simulink model "UAM_controller"  (R2024b)
settings: Solver=FixedStepAuto  StartTime=0.0  StopTime=10.0  RelTol=1e-3
undefined symbols (not defined in the file): control, controlParams, ControlSampleTime, Cruise_a, DiscIntNeverNeededParam, flightState, FWControlParams, FWTrimSpeed, uavParam, w_trim
libraries: slpidlib x41, simulink x7
(part 1 of 6)
settings Model: DataDictionary=UAM_data.sldd  Creator=admin  LastModifiedBy=admin
settings OptimizationCC: DefaultParameterBehavior=Inlined  EnhancedBackFolding=on  PassReuseOutputArgsAs=Individual arguments  ZeroExternalMemoryAtStartup=off  ZeroInternalMemoryAtStartup=off  OptimizeBlockOrder=speed  DifferentSizesBufferReuse=on  OptimizationCustomize=off  EfficientTunableParamExpr=on
settings DebuggingCC: ParameterTunabilityLossMsg=error
settings HardwareCC: ProdBitPerLong=64  ProdLargestAtomicInteger=LongLong  ProdLargestAtomicFloat=Double  ProdLongLongMode=on  ProdHWDeviceType=ARM Compatible->ARM Cortex-A (64-bit)
settings SFSimCC: MATLABDynamicMemAlloc=off
settings RTWCC: Description=Embedded Coder  SystemTargetFile=ert.tlc  TemplateMakefile=ert_default_tmf  Toolchain=Linaro AArch64 Linux v6.3.1
settings CodeAppCC: ForceParamTrailComments=on  IgnoreCustomStorageClasses=off  OperatorAnnotations=on  SimulinkDataObjDesc=on  SFDataObjDesc=on  CustomSymbolStrGlobalVar=CTRL_$N$M  CustomSymbolStrType=CTRL_$N$M_T  CustomSymbolStrField=CTRL_$N$M  CustomSymbolStrFcn=CTRL_$N$M$F  CustomSymbolStrBlkIO=CTRL_rtb_$N$M  CustomSymbolStrTmpVar=CTRL_tmp_$N$M  CustomSymbolStrMacro=CTRL_$N$M_MACRO  InsertBlockDesc=on
settings ERTTargetCC: TargetLangStandard=C99 (ISO)  GenerateSampleERTMain=on  ERTCustomFileTemplate=example_file_process.tlc

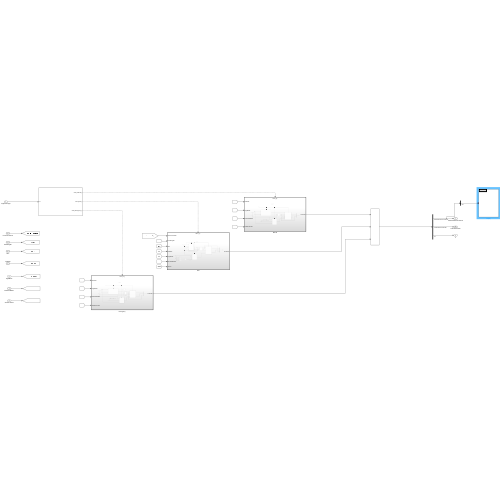
[thumbnail: Simulink's stored preview of the top-level diagram]
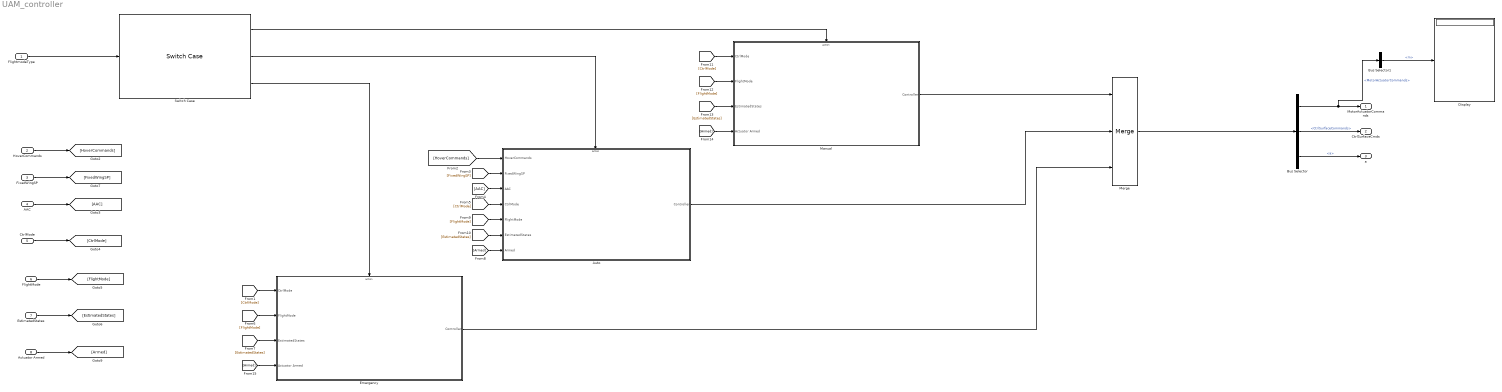
== system UAM_controller ==
  FlightmodeType : Inport  OutDataTypeStr=Enum: FlightModeType
  HoverCommands : Inport  Port=2  OutDataTypeStr=Bus: HoverSPBus
  FixedWingSP : Inport  Port=3  OutDataTypeStr=Bus: FixedWingCommandBus
  AAC : Inport  Port=4  OutDataTypeStr=Bus: AAC
  CtrlMode : Inport  Port=5  OutDataTypeStr=Bus: controlMode
  FlightMode : Inport  Port=6
  EstimatedStates : Inport  Port=7  OutDataTypeStr=Bus: StateBus
  Actuator Armed : Inport  Port=8
  Auto : Subsystem  TreatAsAtomicUnit=on
  Bus Selector : BusSelector  OutputSignals=MotorActuatorCommands,CtrlSurfaceCommands,a
  Bus Selector1 : BusSelector  OutputSignals=m
  Display : Display
  Emergency : Subsystem  TreatAsAtomicUnit=on
  Manual : Subsystem  TreatAsAtomicUnit=on
  Merge : Merge  Inputs=3
  Switch Case : SwitchCase  CaseConditions={FlightModeType.Manual, FlightModeType.Auto, FlightModeType.Emergecny}  ShowDefaultCase=off
  MotorActuatorCommands : Outport  OutDataTypeStr=Bus: FCCData
  CtrlSurfaceCmds : Outport  Port=2  OutDataTypeStr=Bus: FixedWingCtrlBus
  a : Outport  Port=3
  wires:
  FlightmodeType/1 -> Switch Case/1
  CtrlMode/1 -> [CtrlMode]
  HoverCommands/1 -> [HoverCommands]
  EstimatedStates/1 -> [EstimatedStates]
  FlightMode/1 -> [FlightMode]
  AAC/1 -> [AAC]
  FixedWingSP/1 -> [FixedWingSP]
  Actuator Armed/1 -> [Armed]
  [FlightMode] -> Auto/5(FlightMode)
  [Armed] -> Auto/7(" Armed")
  [EstimatedStates] -> Auto/6(EstimatedStates)
  [CtrlMode] -> Auto/4(CtrlMode)
  [AAC] -> Auto/3(AAC)
  [FixedWingSP] -> Auto/2(FixedWingSP)
  [HoverCommands] -> Auto/1(HoverCommands)
  Switch Case/2 -> Auto/Action
  Switch Case/1 -> Manual/Action
  [CtrlMode] -> Manual/1(CtrlMode)
  [FlightMode] -> Manual/2(FlightMode)
  [EstimatedStates] -> Manual/3(EstimatedStates)
  [Armed] -> Manual/4(Actuator Armed)
  [Armed] -> Emergency/4(Actuator Armed)
  [FlightMode] -> Emergency/2(FlightMode)
  [EstimatedStates] -> Emergency/3(EstimatedStates)
  [CtrlMode] -> Emergency/1(CtrlMode)
  Switch Case/3 -> Emergency/Action
  Manual/1(Controller) -> Merge/1
  Merge/1 -> Bus Selector/1
  Bus Selector/1 -> Bus Selector1/1, MotorActuatorCommands/1  "<MotorActuatorCommands>"
  Bus Selector/2 -> CtrlSurfaceCmds/1  "<CtrlSurfaceCommands>"
  Bus Selector/3 -> a/1  "<a>"
  Auto/1(Controller) -> Merge/2
  Emergency/1(Controller) -> Merge/3
  Bus Selector1/1 -> Display/1  "<m>"

== system UAM_controller/Auto ==
  HoverCommands : Inport  OutDataTypeStr=Bus: HoverSPBus
  FixedWingSP : Inport  Port=2
  AAC : Inport  Port=3
  CtrlMode : Inport  Port=4
  FlightMode : Inport  Port=5
  EstimatedStates : Inport  Port=6
  " Armed" : Inport  Port=7
  Action Port : ActionPort  ActionPortLabel=case [ 1 ]:
  Blend Scheduler : Subsystem
  Bus Creator : BusCreator  Inputs=3  OutDataTypeStr=Bus: controller
  Bus Selector2 : BusSelector  OutputSignals=inTransition,TransitionCondition,BackTransitionCondition,TransitionStep
  Fixed Wing Controller : Subsystem  TreatAsAtomicUnit=on  VariantControl=Fixed Wing Controller
  Manual Control : Subsystem
  Multicopter Controller : Subsystem  TreatAsAtomicUnit=on
  Scheduler : Subsystem  SystemSampleTime=0.005
  Controller : Outport
  wires:
  Scheduler/1(MotorActuatorCommands) -> Bus Creator/1  "MotorActuatorCommands"
  Manual Control/1(AERT) -> Fixed Wing Controller/5(AERT)
  Scheduler/2(CtrlSurfaceCommands) -> Bus Creator/2  "CtrlSurfaceCommands"
  Fixed Wing Controller/1(Actuator) -> Scheduler/3(FixedWingActuators)
  Blend Scheduler/2(alpha) -> Bus Creator/3  "a"
  Multicopter Controller/1(MixerCommands) -> Blend Scheduler/3(MixerCommands)
  AAC/1 -> Fixed Wing Controller/3(AAC SP)
  FixedWingSP/1 -> Fixed Wing Controller/4(FixedWingSP)
  [InTransition] -> Multicopter Controller/3(InTransition)
  " Armed"/1 -> Fixed Wing Controller/Enable, Scheduler/Enable, Multicopter Controller/Enable
  HoverCommands/1 -> Multicopter Controller/1(Hover Commands)
  EstimatedStates/1 -> Fixed Wing Controller/1(States), Blend Scheduler/2(States), Multicopter Controller/2(States)
  FlightMode/1 -> Multicopter Controller/4(FlightMode), Blend Scheduler/1(FlightMode)
  Bus Selector2/2 -> [TransitionDone]  "<TransitionCondition>"
  CtrlMode/1 -> Fixed Wing Controller/2(Control Mode), Bus Selector2/1
  Bus Selector2/1 -> [InTransition]  "<inTransition>"
  Bus Selector2/3 -> [BackTransitionDone]  "<BackTransitionCondition>"
  Bus Creator/1 -> Controller/1
  Blend Scheduler/3(FlightState) -> Scheduler/2(FlightState)
  [InTransition] -> Fixed Wing Controller/6(In1)
  Bus Selector2/4 -> [TransitionStep]  "<TransitionStep>"
  Blend Scheduler/1(MotorCommands) -> Scheduler/1(MotorCommands)

== system UAM_controller/Emergency ==
  CtrlMode : Inport  OutDataTypeStr=Bus: controlMode
  FlightMode : Inport  Port=2
  EstimatedStates : Inport  Port=3  OutDataTypeStr=Bus: StateBus
  Actuator Armed : Inport  Port=4
  Action Port : ActionPort  ActionPortLabel=case [ 2 ]:
  Blend Scheduler : Subsystem
  Bus Creator : BusCreator  Inputs=3  OutDataTypeStr=Bus: controller
  Bus Selector : BusSelector  OutputSignals=TransitionCondition,BackTransitionCondition
  Bus Selector1 : BusSelector  OutputSignals=RC
  Display : Display
  FixedWing Controller : Subsystem  TreatAsAtomicUnit=on  VariantControl=Fixed Wing Controller
  Scheduler : Subsystem  SystemSampleTime=0.005
  multicopter Controller : Subsystem  TreatAsAtomicUnit=on
  Controller : Outport
  wires:
  Blend Scheduler/1(alpha) -> Bus Creator/3, Scheduler/2(BlendingSchedule)  "a"
  [TransitionDone] -> Scheduler/4(TransitionDone)
  EstimatedStates/1 -> FixedWing Controller/1(States), Blend Scheduler/2(States), multicopter Controller/2(States), Bus Selector1/1
  FixedWing Controller/1(Actuator) -> Scheduler/6(FixedWingActuators)
  Bus Selector1/1 -> multicopter Controller/1(RC), FixedWing Controller/3(RC)  "<RC>"
  [BackTransitionDone] -> Scheduler/5(BackTransitionDone)
  Bus Selector/2 -> [BackTransitionDone]  "<BackTransitionCondition>"
  FlightMode/1 -> Blend Scheduler/1(FlightMode)
  Bus Selector/1 -> [TransitionDone]  "<TransitionCondition>"
  Actuator Armed/1 -> Scheduler/Enable, FixedWing Controller/Enable, multicopter Controller/Enable
  CtrlMode/1 -> Bus Selector/1, FixedWing Controller/2(Control Mode)
  Blend Scheduler/2(FlightState) -> Scheduler/3(FlightState)
  multicopter Controller/1(MixerCommands) -> Display/1, Scheduler/1(MotorCommands)
  Scheduler/1(MotorActuatorCommands) -> Bus Creator/1  "MotorActuatorCommands"
  Scheduler/2(CtrlSurfaceCommands) -> Bus Creator/2  "CtrlSurfaceCommands"
  Bus Creator/1 -> Controller/1

== system UAM_controller/Manual ==
  CtrlMode : Inport  OutDataTypeStr=Bus: controlMode
  FlightMode : Inport  Port=2
  EstimatedStates : Inport  Port=3  OutDataTypeStr=Bus: StateBus
  Actuator Armed : Inport  Port=4
  Action Port : ActionPort  ActionPortLabel=case [ 0 ]:
  Blend Scheduler : Subsystem
  Bus Creator : BusCreator  Inputs=3  OutDataTypeStr=Bus: controller
  Bus Selector : BusSelector  OutputSignals=TransitionCondition,BackTransitionCondition
  Bus Selector1 : BusSelector  OutputSignals=RC
  FixedWing Controller : Subsystem  TreatAsAtomicUnit=on  VariantControl=Fixed Wing Controller
  Scheduler : Subsystem  SystemSampleTime=0.005
  multicopter Controller : Subsystem  TreatAsAtomicUnit=on
  Controller : Outport
  wires:
  Blend Scheduler/1(alpha) -> Bus Creator/3, Scheduler/2(BlendingSchedule)  "a"
  [TransitionDone] -> Scheduler/4(TransitionDone)
  EstimatedStates/1 -> FixedWing Controller/1(States), Blend Scheduler/2(States), multicopter Controller/2(States), Bus Selector1/1
  FixedWing Controller/1(Actuator) -> Scheduler/6(FixedWingActuators)
  Bus Selector1/1 -> multicopter Controller/1(RC), FixedWing Controller/3(RC)  "<RC>"
  [BackTransitionDone] -> Scheduler/5(BackTransitionDone)
  Bus Selector/2 -> [BackTransitionDone]  "<BackTransitionCondition>"
  FlightMode/1 -> Blend Scheduler/1(FlightMode)
  Bus Selector/1 -> [TransitionDone]  "<TransitionCondition>"
  Actuator Armed/1 -> Scheduler/Enable, FixedWing Controller/Enable, multicopter Controller/Enable
  CtrlMode/1 -> Bus Selector/1, FixedWing Controller/2(Control Mode)
  Blend Scheduler/2(FlightState) -> Scheduler/3(FlightState)
  multicopter Controller/1(MixerCommands) -> Scheduler/1(MotorCommands)
  Scheduler/1(MotorActuatorCommands) -> Bus Creator/1  "MotorActuatorCommands"
  Scheduler/2(CtrlSurfaceCommands) -> Bus Creator/2  "CtrlSurfaceCommands"
  Bus Creator/1 -> Controller/1

== system UAM_controller/Auto/Blend Scheduler ==
  note: Forward Transition Tilt Mode Manager
  FlightMode : Inport
  States : Inport  Port=2
  MixerCommands : Inport  Port=3
  BTalpha : Subsystem  TreatAsAtomicUnit=on
  Bus Creator : BusCreator  Inputs=5
  Bus Selector1 : BusSelector  OutputSignals=w_phi,w_theta,w_psi,w_z
  Constant : Constant  Value=flightState.Transition
  Constant2 : Constant  Value=0.25*uavParam.geom.mass*9.81
  Constant3 : Constant  Value=FWTrimSpeed
  Constant4 : Constant  Value=FWTrimSpeed
  Constant5 : Constant
  Constant6 : Constant  Value=78.54
  Constant7 : Constant
  Demux : Demux
  FTalpha : Subsystem
  Gain3 : Gain  Gain=0
  Mux : Mux
  Product1 : Product
  Product2 : Product
  Product3 : Product
  Relational Operator : RelationalOperator  Operator===  OutDataTypeStr=boolean  RndMeth=Simplest  InputSameDT=off
  Subtract : Sum  Inputs=+-
  Subtract1 : Sum  Inputs=+-
  Sum1 : Sum  Inputs=|++
  Sum3 : Sum  Inputs=|+-
  Switch : Switch  Criteria=u2 > Threshold  SaturateOnIntegerOverflow=off  InputSameDT=off
  Switch1 : Switch  Criteria=u2 > Threshold  SaturateOnIntegerOverflow=off  InputSameDT=off
  MotorCommands : Outport
  alpha : Outport  Port=2
  FlightState : Outport  Port=3
  wires:
  FlightMode/1 -> Relational Operator/1, FlightState/1
  Relational Operator/1 -> [trigger]
  Bus Selector1/4 -> Sum1/1  "<w_z>"
  Constant2/1 -> Sum1/2
  [liftblending] -> Product2/2
  Mux/1 -> Product2/1
  MixerCommands/1 -> Bus Selector1/1
  Bus Selector1/1 -> Mux/1  "<w_phi>"
  Bus Selector1/2 -> Mux/2  "<w_theta>"
  Bus Selector1/3 -> Mux/3  "<w_psi>"
  Sum1/1 -> Mux/4  "w_z"
  Product2/1 -> Demux/1
  Demux/1 -> Bus Creator/1  "w_phi"
  Demux/2 -> Bus Creator/2  "w_theta"
  Demux/3 -> Bus Creator/3  "w_psi"
  Demux/4 -> Bus Creator/4  "w_z"
  Bus Creator/1 -> MotorCommands/1
  Constant6/1 -> Product1/1
  States/1 -> FTalpha/1(States), BTalpha/1(States)
  Switch/1 -> [liftblending], Subtract1/2
  FTalpha/1(alpha) -> Switch/1
  BTalpha/1(alpha) -> Switch/3
  [trigger] -> Switch/2
  Product1/1 -> Sum3/2
  Sum3/1 -> Switch1/1  "cruise"
  [trigger] -> Switch1/2
  Switch1/1 -> Bus Creator/5  "cruise"
  Constant3/1 -> Gain3/1
  Gain3/1 -> Product3/1
  Constant5/1 -> Subtract/1
  [liftblending] -> Subtract/2
  Subtract/1 -> Product3/2
  Product3/1 -> Switch1/3
  Constant7/1 -> Subtract1/1
  Subtract1/1 -> alpha/1
  Constant/1 -> Relational Operator/2
  [liftblending] -> Product1/2
  Constant4/1 -> Sum3/1

== system UAM_controller/Auto/Fixed Wing Controller ==
  States : Inport
  Control Mode : Inport  Port=2
  AAC SP : Inport  Port=3  OutDataTypeStr=Bus: AAC
  FixedWingSP : Inport  Port=4  OutDataTypeStr=Bus: FixedWingCommandBus
  AERT : Inport  Port=5
  In1 : Inport  Port=6
  Actuator Armed : EnablePort
  Subsystem : Subsystem
  Actuator : Outport
  wires:
  States/1 -> Subsystem/1(States)
  Control Mode/1 -> Subsystem/2(Control Mode)
  AAC SP/1 -> Subsystem/3(AAC SP)
  Subsystem/1(Actuator) -> Actuator/1
  AERT/1 -> Subsystem/5(AERT)
  FixedWingSP/1 -> Subsystem/4(FixedWingSP)
  In1/1 -> Subsystem/6(Intransition)

== system UAM_controller/Auto/Manual Control ==
  Bus Creator : BusCreator  Inputs=4
  Constant{,1..3} (4 alike) : Constant  Value=0  SampleTime=-1
  AERT : Outport
  wires:
  Constant/1 -> Bus Creator/1  "aileron"
  Constant1/1 -> Bus Creator/2  "throttle"
  Constant2/1 -> Bus Creator/3  "elevator"
  Constant3/1 -> Bus Creator/4  "rudder"
  Bus Creator/1 -> AERT/1

== system UAM_controller/Auto/Multicopter Controller ==
  note: Prefilter
  Hover Commands : Inport  OutDataTypeStr=Bus: HoverSPBus
  States : Inport  Port=2
  InTransition : Inport  Port=3
  FlightMode : Inport  Port=4
  " Armed" : EnablePort
  Attitude & Altitude controller : Subsystem
  Demux1 : Demux
  Horizontal Position Control : Subsystem  TreatAsAtomicUnit=on
  Merge : Merge
  Merge1 : Merge
  Mux : Mux  Inputs=3
  NOT1 : Logic  Operator=NOT  IconShape=distinctive  AllPortsSameDT=off  OutDataTypeStr=boolean
  Organize Inputs : Subsystem
  transition controller : Subsystem
  MixerCommands : Outport
  wires:
  Organize Inputs/1(MixerCommands) -> MixerCommands/1
  Demux1/1 -> [XRef]
  [State] -> Horizontal Position Control/3(States)
  Demux1/3 -> [ZRef]
  NOT1/1 -> Horizontal Position Control/Enable
  [XRef] -> Horizontal Position Control/1(XRef)
  [YRef] -> Horizontal Position Control/2(YRef)
  InTransition/1 -> [Transition]
  States/1 -> [State]
  Hover Commands/1 -> Demux1/1
  Demux1/4 -> [YawRef]
  Mux/1 -> Attitude & Altitude controller/1(Ref Attitude)
  [State] -> Attitude & Altitude controller/2(States)
  [ZRef] -> Attitude & Altitude controller/3(Z ref)
  [Transition] -> Attitude & Altitude controller/4(InTransition)
  Attitude & Altitude controller/1(Roll torque cmd) -> Organize Inputs/2(commanded phi torque)
  Attitude & Altitude controller/2(Pitch torque Cmd) -> Organize Inputs/3(commanded theta torque)
  Attitude & Altitude controller/4(commanded thrust) -> Organize Inputs/5(commanded thrust)
  FlightMode/1 -> Attitude & Altitude controller/5(FlightMode)
  Attitude & Altitude controller/3(Yaw torque Cmd) -> Organize Inputs/4(commanded psi torque)
  [Transition] -> NOT1/1, transition controller/Enable
  [YawRef] -> Mux/3
  Demux1/2 -> [YRef]
  Merge/1 -> Mux/1
  Merge1/1 -> Mux/2
  transition controller/1(Rollcmd) -> Merge/2
  transition controller/2(Pitchcmd) -> Merge1/2
  Horizontal Position Control/1(Roll Cmd) -> Merge/1
  Horizontal Position Control/2(Pitch Cmd) -> Merge1/1

== system UAM_controller/Auto/Scheduler ==
  MotorCommands : Inport
  FlightState : Inport  Port=2  OutDataTypeStr=Enum: flightState
  FixedWingActuators : Inport  Port=3
  " Armed" : EnablePort
  FixedWingScheduler : Subsystem
  Subsystem : Subsystem
  MotorActuatorCommands : Outport  OutputWhenDisabled=reset  InitialOutput=0
  CtrlSurfaceCommands : Outport  Port=2  OutDataTypeStr=Bus: FixedWingCtrlBus  OutputWhenDisabled=reset  InitialOutput=0  VectorParamsAs1DForOutWhenUnconnected=off
  wires:
  FixedWingScheduler/1(ActuatorControls) -> CtrlSurfaceCommands/1, Subsystem/2(FixedWingActuators)
  FlightState/1 -> Subsystem/1(FlightState), FixedWingScheduler/1(FlightState)
  Subsystem/1(ActuatorControls) -> MotorActuatorCommands/1
  MotorCommands/1 -> Subsystem/3(MotorCommands)
  FixedWingActuators/1 -> FixedWingScheduler/2(FixedWingActuators)

== system UAM_controller/Emergency/Blend Scheduler ==
  FlightMode : Inport
  States : Inport  Port=2
  Constant : Constant  Value=flightState.Transition
  Constant1 : Constant  Value=flightState.BackTransition
  Discrete-Time Integrator : DiscreteIntegrator  gainval=0.01  SampleTime=-1  ICPrevOutput=DiscIntNeverNeededParam  ICPrevScaledInput=DiscIntNeverNeededParam
  Gain : Gain
  Gain1 : Gain  Gain=-1
  Relational Operator : RelationalOperator  Operator===  OutDataTypeStr=boolean  RndMeth=Simplest  InputSameDT=off
  Relational Operator1 : RelationalOperator  Operator===  OutDataTypeStr=boolean  RndMeth=Simplest  InputSameDT=off
  Saturation : Saturate  UpperLimit=1  LowerLimit=0  OutDataTypeStr=double
  Sum : Sum  Inputs=|++
  Terminator : Terminator
  alpha : Outport
  FlightState : Outport  Port=2
  wires:
  FlightMode/1 -> Relational Operator1/1, Relational Operator/1, FlightState/1
  Gain/1 -> Sum/1
  Gain1/1 -> Sum/2
  Sum/1 -> Discrete-Time Integrator/1
  Discrete-Time Integrator/1 -> Saturation/1
  Saturation/1 -> alpha/1  "a"
  States/1 -> Terminator/1
  Constant/1 -> Relational Operator/2
  Relational Operator/1 -> Gain/1
  Constant1/1 -> Relational Operator1/2
  Relational Operator1/1 -> Gain1/1

== system UAM_controller/Emergency/FixedWing Controller ==
  States : Inport
  Control Mode : Inport  Port=2
  RC : Inport  Port=3
  Actuator Armed : EnablePort
  Subsystem : Subsystem
  Actuator : Outport
  wires:
  States/1 -> Subsystem/1(States)
  Control Mode/1 -> Subsystem/2(Control Mode)
  Subsystem/1(Actuator) -> Actuator/1
  RC/1 -> Subsystem/3(RC)

== system UAM_controller/Emergency/Scheduler ==
  MotorCommands : Inport
  BlendingSchedule : Inport  Port=2
  FlightState : Inport  Port=3  OutDataTypeStr=Enum: flightState
  TransitionDone : Inport  Port=4
  BackTransitionDone : Inport  Port=5
  FixedWingActuators : Inport  Port=6  OutDataTypeStr=Bus: FixedWingCtrlBus
  Actuator Armed : EnablePort
  FixedWingScheduler : Subsystem
  Subsystem : Subsystem
  MotorActuatorCommands : Outport  OutputWhenDisabled=reset  InitialOutput=0
  CtrlSurfaceCommands : Outport  Port=2  OutDataTypeStr=Bus: FixedWingCtrlBus  OutputWhenDisabled=reset  InitialOutput=0  VectorParamsAs1DForOutWhenUnconnected=off
  wires:
  FixedWingScheduler/1(ActuatorControls) -> CtrlSurfaceCommands/1, Subsystem/2(FixedWingActuators)
  FlightState/1 -> Subsystem/1(FlightState), FixedWingScheduler/1(FlightState)
  BlendingSchedule/1 -> Subsystem/4(BlendingSchedule)
  Subsystem/1(ActuatorControls) -> MotorActuatorCommands/1
  MotorCommands/1 -> Subsystem/3(MotorCommands)
  FixedWingActuators/1 -> FixedWingScheduler/2(FixedWingActuators)
  TransitionDone/1 -> Subsystem/5(TransitionDone), FixedWingScheduler/3(TransitionDone)
  BackTransitionDone/1 -> Subsystem/6(BackTransitionDone)

== system UAM_controller/Emergency/multicopter Controller ==
  RC : Inport
  States : Inport  Port=2
  Actuator Armed : EnablePort
  Attitude & Altitude controller : Subsystem
  Demux : Demux  Outputs=6
  Mux1 : Mux  Inputs=3
  Organize Inputs : Subsystem
  Terminator : Terminator
  Terminator1 : Terminator
  Terminator2 : Terminator
  MixerCommands : Outport
  wires:
  Demux/6 -> Terminator2/1
  Organize Inputs/1(MixerCommands) -> MixerCommands/1
  Demux/2 -> Organize Inputs/1(forward command), Mux1/2
  Demux/5 -> Terminator1/1
  Attitude & Altitude controller/3(Yaw torque Cmd) -> Organize Inputs/4(commanded psi torque)
  States/1 -> Attitude & Altitude controller/2(States)
  Demux/4 -> Mux1/3
  Attitude & Altitude controller/1(Roll torque cmd) -> Organize Inputs/2(commanded phi torque)
  Attitude & Altitude controller/2(Pitch torque Cmd) -> Organize Inputs/3(commanded theta torque)
  Attitude & Altitude controller/4(commanded thrust) -> Organize Inputs/5(commanded thrust)
  Demux/1 -> Mux1/1
  Mux1/1 -> Attitude & Altitude controller/1(Ref Attitude)
  Demux/3 -> Terminator/1
  RC/1 -> Demux/1

== system UAM_controller/Manual/Blend Scheduler ==
  FlightMode : Inport
  States : Inport  Port=2
  Constant : Constant  Value=flightState.Transition
  Constant1 : Constant  Value=flightState.BackTransition
  Discrete-Time Integrator : DiscreteIntegrator  gainval=0.01  SampleTime=-1  ICPrevOutput=DiscIntNeverNeededParam  ICPrevScaledInput=DiscIntNeverNeededParam
  Gain : Gain
  Gain1 : Gain  Gain=-1
  Relational Operator : RelationalOperator  Operator===  OutDataTypeStr=boolean  RndMeth=Simplest  InputSameDT=off
  Relational Operator1 : RelationalOperator  Operator===  OutDataTypeStr=boolean  RndMeth=Simplest  InputSameDT=off
  Saturation : Saturate  UpperLimit=1  LowerLimit=0  OutDataTypeStr=double
  Sum : Sum  Inputs=|++
  Terminator : Terminator
  alpha : Outport
  FlightState : Outport  Port=2
  wires:
  FlightMode/1 -> Relational Operator1/1, Relational Operator/1, FlightState/1
  Gain/1 -> Sum/1
  Gain1/1 -> Sum/2
  Sum/1 -> Discrete-Time Integrator/1
  Discrete-Time Integrator/1 -> Saturation/1
  Saturation/1 -> alpha/1  "a"
  States/1 -> Terminator/1
  Constant/1 -> Relational Operator/2
  Relational Operator/1 -> Gain/1
  Constant1/1 -> Relational Operator1/2
  Relational Operator1/1 -> Gain1/1

== system UAM_controller/Manual/FixedWing Controller ==
  States : Inport
  Control Mode : Inport  Port=2
  RC : Inport  Port=3
  Actuator Armed : EnablePort
  Subsystem : Subsystem
  Actuator : Outport
  wires:
  States/1 -> Subsystem/1(States)
  Control Mode/1 -> Subsystem/2(Control Mode)
  Subsystem/1(Actuator) -> Actuator/1
  RC/1 -> Subsystem/3(RC)

== system UAM_controller/Manual/Scheduler ==
  MotorCommands : Inport
  BlendingSchedule : Inport  Port=2
  FlightState : Inport  Port=3  OutDataTypeStr=Enum: flightState
  TransitionDone : Inport  Port=4
  BackTransitionDone : Inport  Port=5
  FixedWingActuators : Inport  Port=6  OutDataTypeStr=Bus: FixedWingCtrlBus
  Actuator Armed : EnablePort
  FixedWingScheduler : Subsystem
  Subsystem : Subsystem
  MotorActuatorCommands : Outport  OutputWhenDisabled=reset  InitialOutput=0
  CtrlSurfaceCommands : Outport  Port=2  OutDataTypeStr=Bus: FixedWingCtrlBus  OutputWhenDisabled=reset  InitialOutput=0  VectorParamsAs1DForOutWhenUnconnected=off
  wires:
  FixedWingScheduler/1(ActuatorControls) -> CtrlSurfaceCommands/1, Subsystem/2(FixedWingActuators)
  FlightState/1 -> Subsystem/1(FlightState), FixedWingScheduler/1(FlightState)
  BlendingSchedule/1 -> Subsystem/4(BlendingSchedule)
  Subsystem/1(ActuatorControls) -> MotorActuatorCommands/1
  MotorCommands/1 -> Subsystem/3(MotorCommands)
  FixedWingActuators/1 -> FixedWingScheduler/2(FixedWingActuators)
  TransitionDone/1 -> Subsystem/5(TransitionDone), FixedWingScheduler/3(TransitionDone)
  BackTransitionDone/1 -> Subsystem/6(BackTransitionDone)

== system UAM_controller/Manual/multicopter Controller ==
  RC : Inport
  States : Inport  Port=2
  Actuator Armed : EnablePort
  Attitude & Altitude controller : Subsystem
  Demux : Demux  Outputs=6
  Mux1 : Mux  Inputs=3
  Organize Inputs : Subsystem
  Terminator : Terminator
  Terminator1 : Terminator
  Terminator2 : Terminator
  MixerCommands : Outport
  wires:
  Demux/6 -> Terminator2/1
  Organize Inputs/1(MixerCommands) -> MixerCommands/1
  Demux/2 -> Organize Inputs/1(forward command), Mux1/2
  Demux/5 -> Terminator1/1
  Attitude & Altitude controller/3(Yaw torque Cmd) -> Organize Inputs/4(commanded psi torque)
  States/1 -> Attitude & Altitude controller/2(States)
  Demux/4 -> Mux1/3
  Attitude & Altitude controller/1(Roll torque cmd) -> Organize Inputs/2(commanded phi torque)
  Attitude & Altitude controller/2(Pitch torque Cmd) -> Organize Inputs/3(commanded theta torque)
  Attitude & Altitude controller/4(commanded thrust) -> Organize Inputs/5(commanded thrust)
  Demux/1 -> Mux1/1
  Mux1/1 -> Attitude & Altitude controller/1(Ref Attitude)
  Demux/3 -> Terminator/1
  RC/1 -> Demux/1

== system UAM_controller/Auto/Blend Scheduler/BTalpha ==
  States : Inport
  Bus Selector : BusSelector  OutputSignals=airspeed
  Constant : Constant  Value=65
  Gain : Gain  Gain=1/20
  Saturation : Saturate  UpperLimit=1  LowerLimit=0
  Subtract : Sum  Inputs=+-
  alpha : Outport
  wires:
  Constant/1 -> Subtract/1
  Subtract/1 -> Gain/1
  Gain/1 -> Saturation/1
  Saturation/1 -> alpha/1
  States/1 -> Bus Selector/1
  Bus Selector/1 -> Subtract/2  "<airspeed>"

== system UAM_controller/Auto/Blend Scheduler/FTalpha ==
  States : Inport
  1-a : Sum  Inputs=+-
  Bus Selector : BusSelector  OutputSignals=airspeed
  Constant3 : Constant  Value=35
  Constant5 : Constant  Value=Cruise_a
  Gain3 : Gain  Gain=1/10
  Saturation1 : Saturate  UpperLimit=10  LowerLimit=0
  Sum2 : Sum  Inputs=|+-
  alpha : Outport
  wires:
  1-a/1 -> alpha/1
  Bus Selector/1 -> Sum2/1  "<airspeed>"
  Gain3/1 -> 1-a/2
  Sum2/1 -> Saturation1/1
  Saturation1/1 -> Gain3/1
  Constant3/1 -> Sum2/2
  States/1 -> Bus Selector/1
  Constant5/1 -> 1-a/1

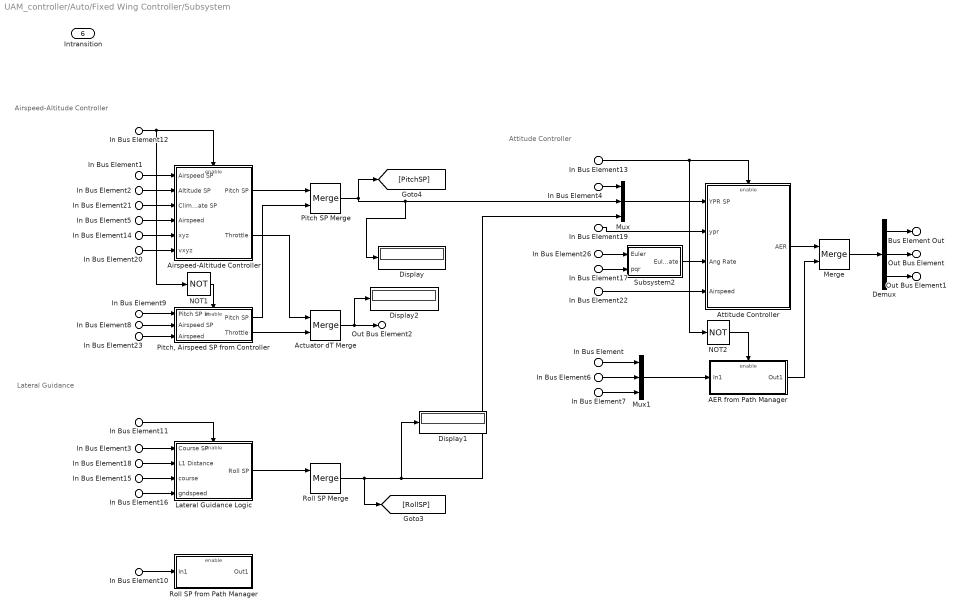
== system UAM_controller/Auto/Fixed Wing Controller/Subsystem ==
  note: Airspeed-Altitude Controller
  note: Lateral Guidance
  note: Attitude Controller
  In Bus Element14 : Inport  PortName=States  Element=Xe
  In Bus Element15 : Inport  PortName=States  Element=course
  In Bus Element17 : Inport  PortName=States  Element=pqr
  In Bus Element5 : Inport  PortName=States  Element=airspeed
  In Bus Element22 : Inport  PortName=States  Element=airspeed
  In Bus Element23 : Inport  PortName=States  Element=airspeed
  In Bus Element19 : Inport  PortName=States  Element=ypr
  In Bus Element16 : Inport  PortName=States  Element=gndspeed
  In Bus Element26 : Inport  PortName=States  Element=Euler
  In Bus Element20 : Inport  PortName=States  Element=Ve_ground
  In Bus Element11 : Inport  Port=2  PortName=Control Mode  Element=lateralGuidance
  In Bus Element12 : Inport  Port=2  PortName=Control Mode  Element=airspeedAltitude
  In Bus Element13 : Inport  Port=2  PortName=Control Mode  Element=attitude
  In Bus Element1 : Inport  Port=3  PortName=AAC SP  Element=airspeed
  In Bus Element2 : Inport  Port=3  PortName=AAC SP  Element=altitude
  In Bus Element18 : Inport  Port=3  PortName=AAC SP  Element=L1
  In Bus Element21 : Inport  Port=3  PortName=AAC SP  Element=course
  In Bus Element3 : Inport  Port=3  PortName=AAC SP  Element=course
  In Bus Element4 : Inport  Port=4  PortName=FixedWingSP  Element=yaw
  In Bus Element9 : Inport  Port=4  PortName=FixedWingSP  Element=pitch
  In Bus Element10 : Inport  Port=4  PortName=FixedWingSP  Element=roll
  In Bus Element8 : Inport  Port=4  PortName=FixedWingSP  Element=airspeed
  In Bus Element : Inport  Port=5  PortName=AERT  Element=aileron
  In Bus Element6 : Inport  Port=5  PortName=AERT  Element=elevator
  In Bus Element7 : Inport  Port=5  PortName=AERT  Element=rudder
  Intransition : Inport  Port=6
  AER from Path Manager : Subsystem  TreatAsAtomicUnit=on
  Actuator dT Merge : Merge
  Airspeed-Altitude Controller : Subsystem
  Attitude Controller : Subsystem
  Demux : Demux  Outputs=3
  Display : Display
  Display1 : Display
  Display2 : Display
  Lateral Guidance Logic : Subsystem
  Merge : Merge
  Mux : Mux  Inputs=3
  Mux1 : Mux  Inputs=3
  NOT1 : Logic  Operator=NOT  IconShape=distinctive  AllPortsSameDT=off  OutDataTypeStr=boolean
  NOT2 : Logic  Operator=NOT  IconShape=distinctive  AllPortsSameDT=off  OutDataTypeStr=boolean
  Pitch SP Merge : Merge
  "Pitch, Airspeed SP from Controller" : Subsystem  TreatAsAtomicUnit=on
  Roll SP Merge : Merge
  Roll SP from Path Manager : Subsystem  TreatAsAtomicUnit=on
  Subsystem2 : Subsystem
  Bus Element Out : Outport  PortName=Actuator  Element=dA
  Out Bus Element : Outport  PortName=Actuator  Element=dE
  Out Bus Element1 : Outport  PortName=Actuator  Element=dR
  Out Bus Element2 : Outport  PortName=Actuator  Element=dT
  wires:
  In Bus Element4/1 -> Mux/1
  Roll SP Merge/1 -> [RollSP], Display1/1, Mux/3
  In Bus Element23/1 -> "Pitch, Airspeed SP from Controller"/3(Airspeed)
  In Bus Element12/1 -> Airspeed-Altitude Controller/Enable, NOT1/1
  In Bus Element3/1 -> Lateral Guidance Logic/1(Course SP)
  Mux1/1 -> AER from Path Manager/1(In1)
  In Bus Element11/1 -> Lateral Guidance Logic/Enable
  Lateral Guidance Logic/1(Roll SP) -> Roll SP Merge/1
  In Bus Element7/1 -> Mux1/3
  Demux/2 -> Out Bus Element/1
  Demux/1 -> Bus Element Out/1
  In Bus Element9/1 -> "Pitch, Airspeed SP from Controller"/1(Pitch SP In)
  Merge/1 -> Demux/1
  In Bus Element18/1 -> Lateral Guidance Logic/2(L1 Distance)
  In Bus Element13/1 -> NOT2/1, Attitude Controller/Enable
  "Pitch, Airspeed SP from Controller"/1(Pitch SP) -> Pitch SP Merge/2
  In Bus Element20/1 -> Airspeed-Altitude Controller/6(vxyz)
  Pitch SP Merge/1 -> Display/1, Mux/2, [PitchSP]
  In Bus Element5/1 -> Airspeed-Altitude Controller/4(Airspeed)
  In Bus Element8/1 -> "Pitch, Airspeed SP from Controller"/2(Airspeed SP)
  In Bus Element15/1 -> Lateral Guidance Logic/3(course)
  Airspeed-Altitude Controller/2(Throttle) -> Actuator dT Merge/1
  In Bus Element21/1 -> Airspeed-Altitude Controller/3(Climb Rate SP)
  In Bus Element1/1 -> Airspeed-Altitude Controller/1(Airspeed SP)
  In Bus Element14/1 -> Airspeed-Altitude Controller/5(xyz)
  In Bus Element22/1 -> Attitude Controller/4(Airspeed)
  In Bus Element2/1 -> Airspeed-Altitude Controller/2(Altitude SP)
  In Bus Element19/1 -> Attitude Controller/2(ypr)
  Mux/1 -> Attitude Controller/1(YPR SP)
  Demux/3 -> Out Bus Element1/1
  In Bus Element26/1 -> Subsystem2/1(Euler)
  Subsystem2/1(Euler Rate) -> Attitude Controller/3(Ang Rate)
  "Pitch, Airspeed SP from Controller"/2(Throttle) -> Actuator dT Merge/2
  Airspeed-Altitude Controller/1(Pitch SP) -> Pitch SP Merge/1
  Attitude Controller/1(AER) -> Merge/1
  AER from Path Manager/1(Out1) -> Merge/2
  In Bus Element/1 -> Mux1/1
  In Bus Element10/1 -> Roll SP from Path Manager/1(In1)
  In Bus Element6/1 -> Mux1/2
  NOT2/1 -> AER from Path Manager/Enable
  In Bus Element17/1 -> Subsystem2/2(pqr)
  Actuator dT Merge/1 -> Display2/1, Out Bus Element2/1
  In Bus Element16/1 -> Lateral Guidance Logic/4(gndspeed)
  NOT1/1 -> "Pitch, Airspeed SP from Controller"/Enable

== system UAM_controller/Auto/Multicopter Controller/Attitude & Altitude controller ==
  Ref Attitude : Inport
  States : Inport  Port=2
  Z ref : Inport  Port=3
  InTransition : Inport  Port=4
  FlightMode : Inport  Port=5
  Altitude Control : Subsystem
      settings: PortSchema="{\"entries\":[{\"content\":{\"sides\":[{\"content\":{\"connectorIds\":[\"In1\",\"In2\",\"In3\"]},\"type\":\"ConnectorPlacement.EquallySpacedRectSide\",\"uuid\":\"0fb78ff2-45dd-421f-94dd-13101ee8437b\"},{\"content\":{\"connectorIds\":[\"Out1\"],\"side\":\"RIGHT\"},\"type\":\"ConnectorPlacement.EquallySpacedRectSide\",\"uuid\":\"b9be60f2-cff5-482a-9939-1f361dc87644\"},{\"content\":{\"side\":\"TOP\"},\"type\":\"ConnectorPlacement.EquallySpacedRectSide\",\"uuid\":\"5554a5d5-69cd-48ac-8e70-482785654dbe\"},{\"content\":{\"connectorIds\":[\"In4\"],\"side\":\"BOTTOM\"},\"type\":\"ConnectorPlacement.EquallySpacedRectSide\",\"uuid\":\"0845aa0b-84ad-4767-a072-4aa91dc150b4\"}]},\"type\":\"ConnectorPlacement.EquallySpacedConnector\",\"uuid\":\"b37117b5-baa1-4c31-85d5-a94c3f794c14\"}],\"packageUris\":[\"http://schema.mathworks.com/mf0/Connector/R2020b\"],\"version\":\"1.0\"}"
  Derivative Gain : Subsystem  VariantControl=AttitudeControl==1
  Roll torque cmd : Outport
  Pitch torque Cmd : Outport  Port=2
  Yaw torque Cmd : Outport  Port=3
  commanded thrust : Outport  Port=4
  wires:
  Altitude Control/1(commanded thrust) -> commanded thrust/1
  Derivative Gain/1(Roll torque cmd) -> Roll torque cmd/1
  InTransition/1 -> Altitude Control/3(InTransition)
  Derivative Gain/2(Pitch torque Cmd) -> Pitch torque Cmd/1
  States/1 -> Derivative Gain/2(States), Altitude Control/1(States)
  Derivative Gain/3(Yaw torque Cmd) -> Yaw torque Cmd/1
  Z ref/1 -> Altitude Control/2(Z ref)
  FlightMode/1 -> Altitude Control/4(FlightMode)
  Ref Attitude/1 -> Derivative Gain/1(Ref Attitude)

== system UAM_controller/Auto/Multicopter Controller/Horizontal Position Control ==
  note: Forward Motion is controlled using Tilt.
      | Lateral Motion occurs using roll.
  XRef : Inport
  YRef : Inport  Port=2
  States : Inport  Port=3
  Enable : EnablePort
  Saturation : Saturate  UpperLimit=0.75  LowerLimit=-0.75
  Saturation1 : Saturate  UpperLimit=1  LowerLimit=-0.75
  Signal Conversion : SignalConversion  OverrideOpt=off
  Signal Conversion1 : SignalConversion  OverrideOpt=off
  XY Controller : Subsystem
  Roll Cmd : Outport
  Pitch Cmd : Outport  Port=2
  wires:
  XRef/1 -> XY Controller/1(X_ref)
  YRef/1 -> XY Controller/2(Y_ref)
  States/1 -> XY Controller/3(States)
  XY Controller/1(Forward cmd) -> Saturation1/1
  XY Controller/2(Sideward Cmd) -> Saturation/1
  Saturation1/1 -> Signal Conversion/1
  Saturation/1 -> Signal Conversion1/1
  Signal Conversion/1 -> Pitch Cmd/1
  Signal Conversion1/1 -> Roll Cmd/1

== system UAM_controller/Auto/Multicopter Controller/Organize Inputs ==
  forward command : Inport
  commanded phi torque : Inport  Port=2
  commanded theta torque : Inport  Port=3
  commanded psi torque : Inport  Port=4
  commanded thrust : Inport  Port=5
  Out Bus Element : Outport  PortName=MixerCommands  Element=w_phi
  Out Bus Element1 : Outport  PortName=MixerCommands  Element=w_theta
  Out Bus Element2 : Outport  PortName=MixerCommands  Element=w_psi
  Out Bus Element3 : Outport  PortName=MixerCommands  Element=w_z
  Out Bus Element4 : Outport  PortName=MixerCommands  Element=l_x
  wires:
  commanded theta torque/1 -> Out Bus Element1/1  "theta"
  commanded psi torque/1 -> Out Bus Element2/1
  commanded thrust/1 -> Out Bus Element3/1
  forward command/1 -> Out Bus Element4/1
  commanded phi torque/1 -> Out Bus Element/1  "phi"

== system UAM_controller/Auto/Multicopter Controller/transition controller ==
  Enable : EnablePort
  Constant : Constant  Value=0
  Constant1 : Constant  Value=0
  Rollcmd : Outport
  Pitchcmd : Outport  Port=2
  wires:
  Constant/1 -> Rollcmd/1
  Constant1/1 -> Pitchcmd/1

== system UAM_controller/Auto/Scheduler/FixedWingScheduler ==
  note: C opyright 2024 The MathWorks, Inc.
  note: Fixed Wing Control Mixer
  FlightState : Inport
  FixedWingActuators : Inport  Port=2  OutDataTypeStr=Bus: FixedWingCtrlBus
  Merge : Merge  Inputs=4
  Switch Case : SwitchCase  CaseConditions={flightState.Hover, flightState.Transition, flightState.FixedWing,flightState.BackTransition}  ShowDefaultCase=off
  Switch Case Action Subsystem : Subsystem  TreatAsAtomicUnit=on
  Switch Case Action Subsystem1 : Subsystem  TreatAsAtomicUnit=on
  Switch Case Action Subsystem2 : Subsystem  TreatAsAtomicUnit=on
  Switch Case Action Subsystem3 : Subsystem  TreatAsAtomicUnit=on
  ActuatorControls : Outport
  wires:
  FlightState/1 -> Switch Case/1
  FixedWingActuators/1 -> Switch Case Action Subsystem2/1(FixedWingActuators), Switch Case Action Subsystem1/1(FixedWingActuators)
  Switch Case/3 -> Switch Case Action Subsystem2/Action
  Switch Case/2 -> Switch Case Action Subsystem1/Action
  Switch Case Action Subsystem3/1(FixedWingControls) -> Merge/4
  Merge/1 -> ActuatorControls/1
  Switch Case Action Subsystem1/1(FixedWingControls) -> Merge/2
  Switch Case/4 -> Switch Case Action Subsystem3/Action
  Switch Case Action Subsystem/1(FixedWingControls) -> Merge/1
  Switch Case/1 -> Switch Case Action Subsystem/Action
  Switch Case Action Subsystem2/1(FixedWingControls) -> Merge/3

== system UAM_controller/Auto/Scheduler/Subsystem ==
  note: C opyright 2024 The MathWorks, Inc.
  note: Multicopter Control Mixer
  FlightState : Inport
  FixedWingActuators : Inport  Port=2
  MotorCommands : Inport  Port=3
  Actuator To Voltage : Subsystem
  Merge : Merge  Inputs=4
  Switch Case : SwitchCase  CaseConditions={flightState.Hover, flightState.Transition, flightState.FixedWing,flightState.BackTransition}  ShowDefaultCase=off
  Switch Case Action Subsystem : Subsystem  TreatAsAtomicUnit=on
  Switch Case Action Subsystem1 : Subsystem  TreatAsAtomicUnit=on
  Switch Case Action Subsystem2 : Subsystem  TreatAsAtomicUnit=on
  Switch Case Action Subsystem3 : Subsystem  TreatAsAtomicUnit=on
  ActuatorControls : Outport  OutDataTypeStr=Bus: FCCData
  wires:
  Switch Case/4 -> Switch Case Action Subsystem3/Action
  MotorCommands/1 -> Switch Case Action Subsystem3/1(MixerCommands), Switch Case Action Subsystem/1(MixerCommands), Switch Case Action Subsystem1/1(MixerCommands)
  FlightState/1 -> Switch Case/1
  Switch Case Action Subsystem3/1(Actuator) -> Merge/4
  FixedWingActuators/1 -> Switch Case Action Subsystem2/1(FixedWingCtrlBus)
  Switch Case/3 -> Switch Case Action Subsystem2/Action
  Switch Case/2 -> Switch Case Action Subsystem1/Action
  Switch Case Action Subsystem1/1(Actuator) -> Merge/2
  Switch Case/1 -> Switch Case Action Subsystem/Action
  Switch Case Action Subsystem2/1(Actuator) -> Merge/3
  Switch Case Action Subsystem/1(Actuator) -> Merge/1
  Merge/1 -> Actuator To Voltage/1(Motor Commands)
  Actuator To Voltage/1(Actuator) -> ActuatorControls/1

== system UAM_controller/Emergency/FixedWing Controller/Subsystem ==
  note: Attitude Controller
  In Bus Element17 : Inport  PortName=States  Element=pqr
  In Bus Element22 : Inport  PortName=States  Element=airspeed
  In Bus Element19 : Inport  PortName=States  Element=ypr
  In Bus Element26 : Inport  PortName=States  Element=Euler
  In Bus Element13 : Inport  Port=2  PortName=Control Mode  Element=attitude
  RC : Inport  Port=3
  Attitude Controller : Subsystem
  Demux : Demux  Outputs=3
  Demux1 : Demux  Outputs=6
  Mux : Mux  Inputs=3
  Subsystem2 : Subsystem
  Terminator1 : Terminator
  Terminator2 : Terminator
  normalization : Subsystem
  normalization1 : Subsystem
  normalization2 : Subsystem
  Bus Element Out : Outport  PortName=Actuator  Element=dA
  Out Bus Element : Outport  PortName=Actuator  Element=dE
  Out Bus Element1 : Outport  PortName=Actuator  Element=dR
  Out Bus Element2 : Outport  PortName=Actuator  Element=dT
  wires:
  Demux/2 -> Out Bus Element/1
  Demux/1 -> Bus Element Out/1
  In Bus Element13/1 -> Attitude Controller/Enable
  In Bus Element22/1 -> Attitude Controller/4(Airspeed)
  In Bus Element19/1 -> Attitude Controller/2(ypr)
  Mux/1 -> Attitude Controller/1(YPR SP)
  Demux/3 -> Out Bus Element1/1
  In Bus Element26/1 -> Subsystem2/1(Euler)
  Subsystem2/1(Euler Rate) -> Attitude Controller/3(Ang Rate)
  Attitude Controller/1(AER) -> Demux/1
  In Bus Element17/1 -> Subsystem2/2(pqr)
  RC/1 -> Demux1/1
  Demux1/1 -> normalization1/1(In1)  "roll"
  Demux1/2 -> normalization2/1(In1)  "pitch"
  Demux1/3 -> Out Bus Element2/1  "throttle"
  Demux1/4 -> normalization/1(In1)  "yaw"
  Demux1/5 -> Terminator1/1
  normalization/1(Out1) -> Mux/1
  normalization1/1(Out1) -> Mux/2
  normalization2/1(Out1) -> Mux/3
  Demux1/6 -> Terminator2/1

== system UAM_controller/Emergency/Scheduler/FixedWingScheduler ==
  note: C opyright 2024 The MathWorks, Inc.
  note: Fixed Wing Control Mixer
  FlightState : Inport
  FixedWingActuators : Inport  Port=2  OutDataTypeStr=Bus: FixedWingCtrlBus
  TransitionDone : Inport  Port=3
  Merge : Merge  Inputs=4
  Switch Case : SwitchCase  CaseConditions={flightState.Hover, flightState.Transition, flightState.FixedWing,flightState.BackTransition}  ShowDefaultCase=off
  Switch Case Action Subsystem : Subsystem  TreatAsAtomicUnit=on
  Switch Case Action Subsystem1 : Subsystem  TreatAsAtomicUnit=on
  Switch Case Action Subsystem2 : Subsystem  TreatAsAtomicUnit=on
  Switch Case Action Subsystem3 : Subsystem  TreatAsAtomicUnit=on
  ActuatorControls : Outport  OutDataTypeStr=Bus: FixedWingCtrlBus
  wires:
  FlightState/1 -> Switch Case/1
  FixedWingActuators/1 -> Switch Case Action Subsystem2/1(FixedWingActuators), Switch Case Action Subsystem1/1(FixedWingActuators)
  Switch Case/3 -> Switch Case Action Subsystem2/Action
  Switch Case/2 -> Switch Case Action Subsystem1/Action
  TransitionDone/1 -> Switch Case Action Subsystem1/2(TransitionDone)
  Switch Case Action Subsystem3/1(FixedWingControls) -> Merge/4
  Merge/1 -> ActuatorControls/1
  Switch Case Action Subsystem1/1(FixedWingControls) -> Merge/2
  Switch Case/4 -> Switch Case Action Subsystem3/Action
  Switch Case Action Subsystem/1(FixedWingControls) -> Merge/1
  Switch Case/1 -> Switch Case Action Subsystem/Action
  Switch Case Action Subsystem2/1(FixedWingControls) -> Merge/3

== system UAM_controller/Emergency/Scheduler/Subsystem ==
  note: C opyright 2024 The MathWorks, Inc.
  note: Multicopter Control Mixer
  FlightState : Inport
  FixedWingActuators : Inport  Port=2
  MotorCommands : Inport  Port=3
  BlendingSchedule : Inport  Port=4
  TransitionDone : Inport  Port=5
  BackTransitionDone : Inport  Port=6
  Actuator To Voltage : Subsystem
  Merge : Merge  Inputs=4
  Switch Case : SwitchCase  CaseConditions={flightState.Hover, flightState.Transition, flightState.FixedWing,flightState.BackTransition}  ShowDefaultCase=off
  Switch Case Action Subsystem : Subsystem  TreatAsAtomicUnit=on
  Switch Case Action Subsystem1 : Subsystem  TreatAsAtomicUnit=on
  Switch Case Action Subsystem2 : Subsystem  TreatAsAtomicUnit=on
  Switch Case Action Subsystem3 : Subsystem  TreatAsAtomicUnit=on
  ActuatorControls : Outport  OutDataTypeStr=Bus: FCCData
  wires:
  Switch Case/4 -> Switch Case Action Subsystem3/Action
  MotorCommands/1 -> Switch Case Action Subsystem3/2(MixerCommands), Switch Case Action Subsystem/1(MixerCommands), Switch Case Action Subsystem1/2(MixerCommands)
  FlightState/1 -> Switch Case/1
  Switch Case Action Subsystem/1(Actuator) -> Merge/1
  Switch Case Action Subsystem3/1(Actuator) -> Merge/4
  FixedWingActuators/1 -> Switch Case Action Subsystem2/1(FixedWingCtrlBus), Switch Case Action Subsystem1/3(FixedWing)
  Switch Case/3 -> Switch Case Action Subsystem2/Action
  TransitionDone/1 -> Switch Case Action Subsystem1/4(TransitionDone)
  Switch Case/2 -> Switch Case Action Subsystem1/Action
  Switch Case Action Subsystem1/1(Actuator) -> Merge/2
  BlendingSchedule/1 -> Switch Case Action Subsystem1/1(BlendingSchedule), Switch Case Action Subsystem3/1(BlendingSchedule)
  Switch Case/1 -> Switch Case Action Subsystem/Action
  BackTransitionDone/1 -> Switch Case Action Subsystem3/3(BackTransitionDone)
  Switch Case Action Subsystem2/1(Actuator) -> Merge/3
  Actuator To Voltage/1(Actuator) -> ActuatorControls/1
  Merge/1 -> Actuator To Voltage/1(Motor Commands)

== system UAM_controller/Emergency/multicopter Controller/Attitude & Altitude controller ==
  Ref Attitude : Inport
  States : Inport  Port=2
  Bias : Bias  Bias=-1500  SaturateOnIntegerOverflow=off
  Bus Selector : BusSelector  OutputSignals=RC
  Derivative Gain : Subsystem  VariantControl=AttitudeControl==1
  Display : Display
  Gain : Gain  Gain=1/500
  Selector : Selector  InputPortWidth=6  IndexOptions=Index vector (dialog)  Indices=3  OutputSizes=1
  Roll torque cmd : Outport
  Pitch torque Cmd : Outport  Port=2
  Yaw torque Cmd : Outport  Port=3
  commanded thrust : Outport  Port=4
  wires:
  Derivative Gain/1(Roll torque cmd) -> Roll torque cmd/1
  Derivative Gain/2(Pitch torque Cmd) -> Pitch torque Cmd/1
  States/1 -> Bus Selector/1, Derivative Gain/2(States)
  Derivative Gain/3(Yaw torque Cmd) -> Yaw torque Cmd/1
  Ref Attitude/1 -> Derivative Gain/1(Ref Attitude)
  Bus Selector/1 -> Selector/1  "<RC>"
  Selector/1 -> Bias/1
  Bias/1 -> Gain/1
  Gain/1 -> Display/1, commanded thrust/1

== system UAM_controller/Emergency/multicopter Controller/Organize Inputs ==
  forward command : Inport
  commanded phi torque : Inport  Port=2
  commanded theta torque : Inport  Port=3
  commanded psi torque : Inport  Port=4
  commanded thrust : Inport  Port=5
  Display{,1..3} (4 alike) : Display
  Out Bus Element : Outport  PortName=MixerCommands  Element=w_phi
  Out Bus Element1 : Outport  PortName=MixerCommands  Element=w_theta
  Out Bus Element2 : Outport  PortName=MixerCommands  Element=w_psi
  Out Bus Element3 : Outport  PortName=MixerCommands  Element=w_z
  Out Bus Element4 : Outport  PortName=MixerCommands  Element=l_x
  wires:
  commanded theta torque/1 -> Display2/1, Out Bus Element1/1  "theta"
  commanded psi torque/1 -> Display1/1, Out Bus Element2/1
  commanded thrust/1 -> Display/1, Out Bus Element3/1
  forward command/1 -> Out Bus Element4/1
  commanded phi torque/1 -> Display3/1, Out Bus Element/1  "phi"

== system UAM_controller/Manual/FixedWing Controller/Subsystem ==
  note: Attitude Controller
  In Bus Element17 : Inport  PortName=States  Element=pqr
  In Bus Element22 : Inport  PortName=States  Element=airspeed
  In Bus Element19 : Inport  PortName=States  Element=ypr
  In Bus Element26 : Inport  PortName=States  Element=Euler
  In Bus Element13 : Inport  Port=2  PortName=Control Mode  Element=attitude
  RC : Inport  Port=3
  Attitude Controller : Subsystem
  Demux : Demux  Outputs=3
  Demux1 : Demux  Outputs=6
  Mux : Mux  Inputs=3
  Subsystem2 : Subsystem
  Terminator1 : Terminator
  Terminator2 : Terminator
  normalization : Subsystem
  normalization1 : Subsystem
  normalization2 : Subsystem
  Bus Element Out : Outport  PortName=Actuator  Element=dA
  Out Bus Element : Outport  PortName=Actuator  Element=dE
  Out Bus Element1 : Outport  PortName=Actuator  Element=dR
  Out Bus Element2 : Outport  PortName=Actuator  Element=dT
  wires:
  Demux/2 -> Out Bus Element/1
  Demux/1 -> Bus Element Out/1
  In Bus Element13/1 -> Attitude Controller/Enable
  In Bus Element22/1 -> Attitude Controller/4(Airspeed)
  In Bus Element19/1 -> Attitude Controller/2(ypr)
  Mux/1 -> Attitude Controller/1(YPR SP)
  Demux/3 -> Out Bus Element1/1
  In Bus Element26/1 -> Subsystem2/1(Euler)
  Subsystem2/1(Euler Rate) -> Attitude Controller/3(Ang Rate)
  Attitude Controller/1(AER) -> Demux/1
  In Bus Element17/1 -> Subsystem2/2(pqr)
  RC/1 -> Demux1/1
  Demux1/1 -> normalization1/1(In1)  "roll"
  Demux1/2 -> normalization2/1(In1)  "pitch"
  Demux1/3 -> Out Bus Element2/1  "throttle"
  Demux1/4 -> normalization/1(In1)  "yaw"
  Demux1/5 -> Terminator1/1
  normalization/1(Out1) -> Mux/1
  normalization1/1(Out1) -> Mux/2
  normalization2/1(Out1) -> Mux/3
  Demux1/6 -> Terminator2/1

== system UAM_controller/Manual/Scheduler/FixedWingScheduler ==
  note: C opyright 2024 The MathWorks, Inc.
  note: Fixed Wing Control Mixer
  FlightState : Inport
  FixedWingActuators : Inport  Port=2  OutDataTypeStr=Bus: FixedWingCtrlBus
  TransitionDone : Inport  Port=3
  Merge : Merge  Inputs=4
  Switch Case : SwitchCase  CaseConditions={flightState.Hover, flightState.Transition, flightState.FixedWing,flightState.BackTransition}  ShowDefaultCase=off
  Switch Case Action Subsystem : Subsystem  TreatAsAtomicUnit=on
  Switch Case Action Subsystem1 : Subsystem  TreatAsAtomicUnit=on
  Switch Case Action Subsystem2 : Subsystem  TreatAsAtomicUnit=on
  Switch Case Action Subsystem3 : Subsystem  TreatAsAtomicUnit=on
  ActuatorControls : Outport  OutDataTypeStr=Bus: FixedWingCtrlBus
  wires:
  FlightState/1 -> Switch Case/1
  FixedWingActuators/1 -> Switch Case Action Subsystem2/1(FixedWingActuators), Switch Case Action Subsystem1/1(FixedWingActuators)
  Switch Case/3 -> Switch Case Action Subsystem2/Action
  Switch Case/2 -> Switch Case Action Subsystem1/Action
  TransitionDone/1 -> Switch Case Action Subsystem1/2(TransitionDone)
  Switch Case Action Subsystem3/1(FixedWingControls) -> Merge/4
  Merge/1 -> ActuatorControls/1
  Switch Case Action Subsystem1/1(FixedWingControls) -> Merge/2
  Switch Case/4 -> Switch Case Action Subsystem3/Action
  Switch Case Action Subsystem/1(FixedWingControls) -> Merge/1
  Switch Case/1 -> Switch Case Action Subsystem/Action
  Switch Case Action Subsystem2/1(FixedWingControls) -> Merge/3
